simulink model "test_cpg_auto"  (R2022a)
settings: Solver=VariableStepAuto  StartTime=0.0  StopTime=10.0  RelTol=1e-3
values from neighbouring files (symbols this model uses):
  dfm = dfm_def    (= 0)    [autotest.m]    (also in flCurvesODEModel.m; freqStat.m = fieldOrDefault(params, "dfm", 0.0))
  dsm = values(i)    [autotest.m]    (also in flCurvesODEModel.m = -0.5; freqStat.m = fieldOrDefault(params, "dsm", -0.5))
  dsp = dsp_def    (= 0.5)    [autotest.m]    (also in flCurvesODEModel.m; freqStat.m = fieldOrDefault(params, "dsp", 0.5))
  dup = dup_def    (= -0.5)    [autotest.m]    (also in flCurvesODEModel.m; freqStat.m = fieldOrDefault(params, "dup", -0.5))
  gfm = gfm_def    (= -2)    [autotest.m]    (also in flCurvesODEModel.m; freqStat.m = fieldOrDefault(params, "gfm", -2))
  gsm = gsm_def    (= -4)    [autotest.m]    (also in flCurvesODEModel.m = -2; freqStat.m = fieldOrDefault(params, "gsm", -4))
  gsp = gsp_def    (= 6)    [autotest.m]    (also in flCurvesODEModel.m; freqStat.m = fieldOrDefault(params, "gsp", 6))
  gup = gup_def    (= 5)    [autotest.m]    (also in flCurvesODEModel.m = 0; freqStat.m = fieldOrDefault(params, "gup", 5))
  Iapp = timeseries(Iin,time)    [autotest.m]    (also in flCurvesODEModel.m = @(t) I0; freqStat.m = timeseries(Iapp_val, time); tests.m = -1)
  sampleTime = 0.0001    [autotest.m]    (also in freqStat.m = fieldOrDefault(params, "sampleTime", 0.0001))
undefined symbols (not defined in the file or in its folder): dsyn, gsyn, noisePwr
libraries: simulink x2
settings Model: Creator=chris  LastModifiedBy=chris

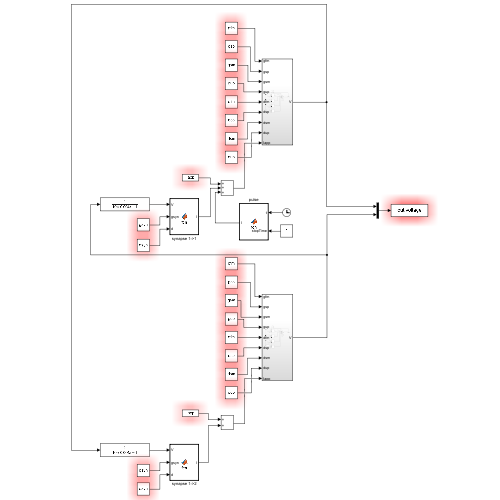
[thumbnail: Simulink's stored preview of the top-level diagram]
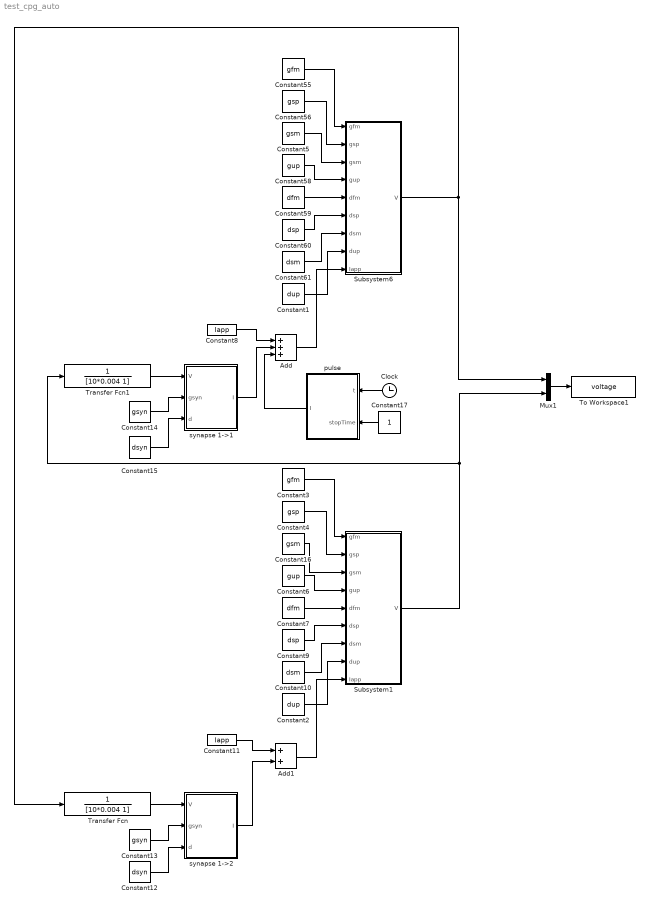
== system test_cpg_auto ==
  Add : Sum  Inputs=+++
  Add1 : Sum
  Clock : Clock
  Constant1 : Constant  Value=dup
  Constant10 : Constant  Value=dsm
  Constant11 : Constant  Value=Iapp
  Constant12 : Constant  Value=dsyn
  Constant13 : Constant  Value=gsyn
  Constant14 : Constant  Value=gsyn
  Constant15 : Constant  Value=dsyn
  Constant16 : Constant  Value=gsm
  Constant17 : Constant
  Constant2 : Constant  Value=dup
  Constant3 : Constant  Value=gfm
  Constant4 : Constant  Value=gsp
  Constant5 : Constant  Value=gsm
  Constant55 : Constant  Value=gfm
  Constant56 : Constant  Value=gsp
  Constant58 : Constant  Value=gup
  Constant59 : Constant  Value=dfm
  Constant6 : Constant  Value=gup
  Constant60 : Constant  Value=dsp
  Constant61 : Constant  Value=dsm
  Constant7 : Constant  Value=dfm
  Constant8 : Constant  Value=Iapp
  Constant9 : Constant  Value=dsp
  Mux1 : Mux  Inputs=2
  Subsystem1 : Subsystem
  Subsystem6 : Subsystem
  To Workspace1 : ToWorkspace  VariableName=voltage  SaveFormat=Structure With Time  SampleTime=sampleTime
  Transfer Fcn : TransferFcn  Denominator=[10*0.004 1]
  Transfer Fcn1 : TransferFcn  Denominator=[10*0.004 1]
  pulse : MATLAB Function  TreatAsAtomicUnit=on
  synapse 1->1 : MATLAB Function  TreatAsAtomicUnit=on
  synapse 1->2 : MATLAB Function  TreatAsAtomicUnit=on
  wires:
  Constant59/1 -> Subsystem6/5(dfm)
  Constant6/1 -> Subsystem1/4(gup)
  Constant9/1 -> Subsystem1/6(dsp)
  Constant55/1 -> Subsystem6/1(gfm)
  synapse 1->1/1(I) -> Add/2
  Add/1 -> Subsystem6/9(Iapp)
  Constant13/1 -> synapse 1->2/2(gsyn)
  Constant3/1 -> Subsystem1/1(gfm)
  Constant10/1 -> Subsystem1/7(dsm)
  Constant14/1 -> synapse 1->1/2(gsyn)
  Constant7/1 -> Subsystem1/5(dfm)
  Transfer Fcn/1 -> synapse 1->2/1(V)
  Constant2/1 -> Subsystem1/8(dup)
  Add1/1 -> Subsystem1/9(Iapp)
  Constant4/1 -> Subsystem1/2(gsp)
  Constant12/1 -> synapse 1->2/3(d)
  Constant11/1 -> Add1/1
  synapse 1->2/1(I) -> Add1/2
  Subsystem1/1(V) -> Mux1/2, Transfer Fcn1/1
  Constant56/1 -> Subsystem6/2(gsp)
  Constant60/1 -> Subsystem6/6(dsp)
  Constant1/1 -> Subsystem6/8(dup)
  Constant61/1 -> Subsystem6/7(dsm)
  Constant58/1 -> Subsystem6/4(gup)
  Constant15/1 -> synapse 1->1/3(d)
  Constant8/1 -> Add/1
  Transfer Fcn1/1 -> synapse 1->1/1(V)
  Subsystem6/1(V) -> Transfer Fcn/1, Mux1/1
  Constant5/1 -> Subsystem6/3(gsm)
  Constant16/1 -> Subsystem1/3(gsm)
  Mux1/1 -> To Workspace1/1
  pulse/1(I) -> Add/3
  Constant17/1 -> pulse/2(stopTime)
  Clock/1 -> pulse/1(t)

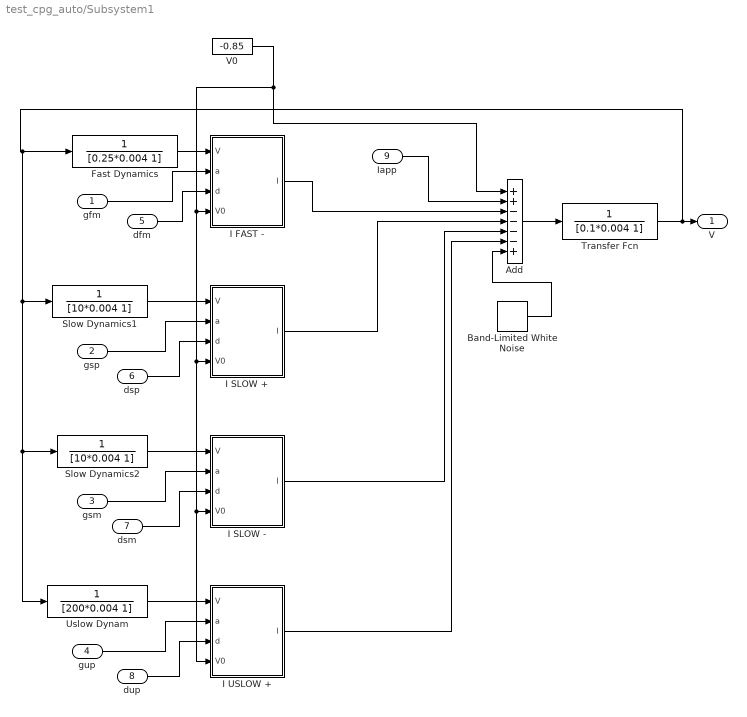
== system test_cpg_auto/Subsystem1 ==
  gfm : Inport
  gsp : Inport  Port=2
  gsm : Inport  Port=3
  gup : Inport  Port=4
  dfm : Inport  Port=5
  dsp : Inport  Port=6
  dsm : Inport  Port=7
  dup : Inport  Port=8
  Iapp : Inport  Port=9
  Add : Sum  Inputs=++----+
  Band-Limited White Noise : simulink/Sources/Band-Limited White Noise  Cov=[noisePwr]  Ts=0.001  seed=floor(rand(1)*250000)
  Fast Dynamics : TransferFcn  Denominator=[0.25*0.004 1]
  I FAST - : MATLAB Function  TreatAsAtomicUnit=on
  I SLOW + : MATLAB Function  TreatAsAtomicUnit=on
  I SLOW - : MATLAB Function  TreatAsAtomicUnit=on
  I USLOW + : MATLAB Function  TreatAsAtomicUnit=on
  Slow Dynamics1 : TransferFcn  Denominator=[10*0.004 1]
  Slow Dynamics2 : TransferFcn  Denominator=[10*0.004 1]
  Transfer Fcn : TransferFcn  Denominator=[0.1*0.004 1]
  Uslow Dynam : TransferFcn  Denominator=[200*0.004 1]
  V0 : Constant  Value=-0.85
  V : Outport
  wires:
  dup/1 -> I USLOW +/3(d)
  gsm/1 -> I SLOW -/2(a)
  dsm/1 -> I SLOW -/3(d)
  gup/1 -> I USLOW +/2(a)
  Iapp/1 -> Add/2
  Uslow Dynam/1 -> I USLOW +/1(V)
  Add/1 -> Transfer Fcn/1
  Slow Dynamics1/1 -> I SLOW +/1(V)
  Slow Dynamics2/1 -> I SLOW -/1(V)
  I FAST -/1(I) -> Add/3
  I USLOW +/1(I) -> Add/6
  V0/1 -> I USLOW +/4(V0), I SLOW -/4(V0), I SLOW +/4(V0), I FAST -/4(V0), Add/1
  dsp/1 -> I SLOW +/3(d)
  gsp/1 -> I SLOW +/2(a)
  dfm/1 -> I FAST -/3(d)
  gfm/1 -> I FAST -/2(a)
  Fast Dynamics/1 -> I FAST -/1(V)
  I SLOW -/1(I) -> Add/5
  Transfer Fcn/1 -> Uslow Dynam/1, Slow Dynamics2/1, Slow Dynamics1/1, Fast Dynamics/1, V/1
  I SLOW +/1(I) -> Add/4
  Band-Limited White Noise/1 -> Add/7

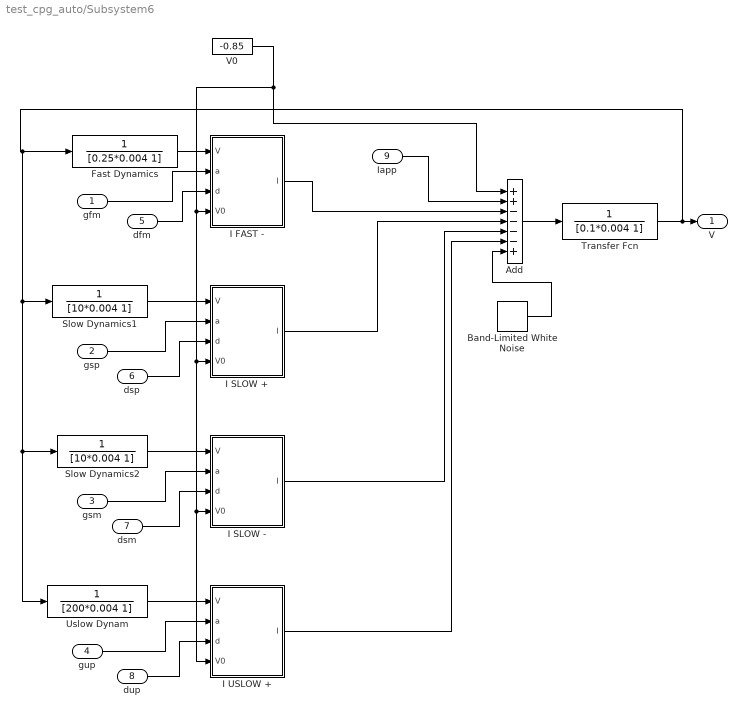
== system test_cpg_auto/Subsystem6 ==
  gfm : Inport
  gsp : Inport  Port=2
  gsm : Inport  Port=3
  gup : Inport  Port=4
  dfm : Inport  Port=5
  dsp : Inport  Port=6
  dsm : Inport  Port=7
  dup : Inport  Port=8
  Iapp : Inport  Port=9
  Add : Sum  Inputs=++----+
  Band-Limited White Noise : simulink/Sources/Band-Limited White Noise  Cov=[noisePwr]  Ts=0.001  seed=floor(rand(1)*250000)
  Fast Dynamics : TransferFcn  Denominator=[0.25*0.004 1]
  I FAST - : MATLAB Function  TreatAsAtomicUnit=on
  I SLOW + : MATLAB Function  TreatAsAtomicUnit=on
  I SLOW - : MATLAB Function  TreatAsAtomicUnit=on
  I USLOW + : MATLAB Function  TreatAsAtomicUnit=on
  Slow Dynamics1 : TransferFcn  Denominator=[10*0.004 1]
  Slow Dynamics2 : TransferFcn  Denominator=[10*0.004 1]
  Transfer Fcn : TransferFcn  Denominator=[0.1*0.004 1]
  Uslow Dynam : TransferFcn  Denominator=[200*0.004 1]
  V0 : Constant  Value=-0.85
  V : Outport
  wires:
  dup/1 -> I USLOW +/3(d)
  gsm/1 -> I SLOW -/2(a)
  dsm/1 -> I SLOW -/3(d)
  gup/1 -> I USLOW +/2(a)
  Iapp/1 -> Add/2
  Uslow Dynam/1 -> I USLOW +/1(V)
  Add/1 -> Transfer Fcn/1
  Slow Dynamics1/1 -> I SLOW +/1(V)
  Slow Dynamics2/1 -> I SLOW -/1(V)
  I FAST -/1(I) -> Add/3
  I USLOW +/1(I) -> Add/6
  V0/1 -> I USLOW +/4(V0), I SLOW -/4(V0), I SLOW +/4(V0), I FAST -/4(V0), Add/1
  dsp/1 -> I SLOW +/3(d)
  gsp/1 -> I SLOW +/2(a)
  dfm/1 -> I FAST -/3(d)
  gfm/1 -> I FAST -/2(a)
  Fast Dynamics/1 -> I FAST -/1(V)
  I SLOW -/1(I) -> Add/5
  Transfer Fcn/1 -> Uslow Dynam/1, Slow Dynamics2/1, Slow Dynamics1/1, Fast Dynamics/1, V/1
  I SLOW +/1(I) -> Add/4
  Band-Limited White Noise/1 -> Add/7

== matlab function test_cpg_auto/Subsystem1/I FAST - ==
  data: V input; I output; a input; d input; V0 input
function I = fcn(V,a,d,V0)

I = a*(tanh(V-d)-tanh(V0-d));

== matlab function test_cpg_auto/Subsystem6/I USLOW + ==
  data: V input; I output; a input; d input; V0 input
function I = fcn(V,a,d,V0)

I = a*(tanh(V-d)-tanh(V0-d));

== matlab function test_cpg_auto/Subsystem1/I SLOW + ==
  data: V input; I output; a input; d input; V0 input
function I = fcn(V,a,d,V0)

I = a*(tanh(V-d)-tanh(V0-d));

== matlab function test_cpg_auto/Subsystem1/I SLOW - ==
  data: V input; I output; a input; d input; V0 input
function I = fcn(V,a,d,V0)

I = a*(tanh(V-d)-tanh(V0-d));

== matlab function test_cpg_auto/Subsystem1/I USLOW + ==
  data: V input; I output; a input; d input; V0 input
function I = fcn(V,a,d,V0)

I = a*(tanh(V-d)-tanh(V0-d));

== matlab function test_cpg_auto/synapse 1->1 ==
  data: V input; I output; gsyn input; d input
function I = fcn(V,gsyn,d)

I = gsyn*(tanh(2*(V-d))+1)/2;

== matlab function test_cpg_auto/pulse ==
  data: t input; I output; stopTime input
function I = fcn(t, stopTime)

if t < stopTime
    I = 3;
else
    I = 0;
end

== matlab function test_cpg_auto/synapse 1->2 ==
  data: V input; I output; gsyn input; d input
function I = fcn(V,gsyn,d)

I = gsyn*(tanh(2*(V-d))+1)/2;

== matlab function test_cpg_auto/Subsystem6/I FAST - ==
  data: V input; I output; a input; d input; V0 input
function I = fcn(V,a,d,V0)

I = a*(tanh(V-d)-tanh(V0-d));

== matlab function test_cpg_auto/Subsystem6/I SLOW + ==
  data: V input; I output; a input; d input; V0 input
function I = fcn(V,a,d,V0)

I = a*(tanh(V-d)-tanh(V0-d));

== matlab function test_cpg_auto/Subsystem6/I SLOW - ==
  data: V input; I output; a input; d input; V0 input
function I = fcn(V,a,d,V0)

I = a*(tanh(V-d)-tanh(V0-d));
